simulink model "cllc_plant"  (R2020b)
settings: Solver=FixedStepDiscrete  StartTime=0.0  StopTime=Inf  FixedStep=stepsize  RelTol=1e-3  EnableMultiTasking=on
values from neighbouring files (symbols this model uses):
  Lm1 = Ln*LrP1    (= 0.00016)    [CLLC_Plant_Parameters.m]
  n = 20.0/9.0    (= 2.22222222222)    [CLLC_Plant_Parameters.m]
  stepsize = 2.0E-7    [cllc_data_lib.sldd]
  var_dir_v2g = 0.0    [cllc_data_lib.sldd]
  var_ref_iout = 18.5    [cllc_data_lib.sldd]
  var_ref_vout = 250.0    [cllc_data_lib.sldd]
libraries: fl_lib x219, ee_lib x151, nesl_utility x117, powerlib_meascontrol x15, eeStairGenerator x1
(part 1 of 8)
settings Model: DataDictionary=cllc_data_lib.sldd  ExtModeTrigDuration=8  Creator=wanikmalwansulami  LastModifiedBy=sgcesuser2
settings SolverCC: AutoInsertRateTranBlk=on  InsertRTBMode=Always
settings DataIOCC: SaveOutput=off  SaveTime=off  ReturnWorkspaceOutputs=off
settings OptimizationCC: DefaultUnderspecifiedDataType=single  EnhancedBackFolding=on  PassReuseOutputArgsAs=Individual arguments  MaxStackSize=1024  OptimizeBlockOrder=speed  DifferentSizesBufferReuse=on  OptimizationCustomize=off  DenormalBehavior=FlushToZero  EfficientTunableParamExpr=on
settings DebuggingCC: ParameterTunabilityLossMsg=error
settings HardwareCC: ProdBitPerChar=16  ProdBitPerInt=16  ProdBitPerPointer=32  ProdBitPerSizeT=32  ProdBitPerPtrDiffT=32  ProdLargestAtomicInteger=Integer  ProdLargestAtomicFloat=None  ProdWordSize=16  ProdLongLongMode=on  ProdHWDeviceType=Texas Instruments->C2000
settings SFSimCC: MATLABDynamicMemAlloc=off  CustomCodeUndefinedFunction=UseInterfaceOnly
settings RTWCC: Description=Embedded Coder  SystemTargetFile=ert.tlc  HardwareBoard=TI Piccolo F2807x  TemplateMakefile=ert_default_tmf  Toolchain=Texas Instruments Code Composer Studio (C2000)  PortableWordSizes=on
settings CodeAppCC: ForceParamTrailComments=on  IgnoreCustomStorageClasses=off  OperatorAnnotations=on  SimulinkDataObjDesc=on  SFDataObjDesc=on  InsertBlockDesc=on
settings ERTTargetCC: CodeReplacementLibrary=TI C28x  CombineOutputUpdateFcns=off  SupportContinuousTime=on  SupportNonInlinedSFcns=on  ExtModeStaticAllocSize=2000
settings SimscapeCC: SimscapeLogSimulationStatistics=on  SimscapeLogLimitData=off

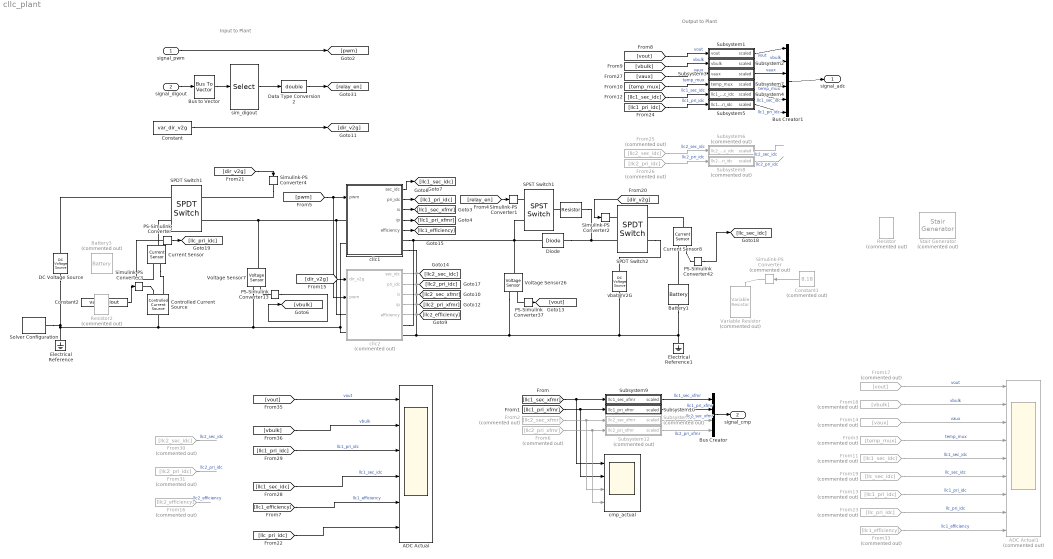
== system cllc_plant ==
  note: Input to Plant
  note: Output to Plant
  signal_pwm : Inport
  signal_digout : Inport  Port=2
  " " : ee_lib/Passive/Resistor  R=0.5e-3 Ohm  R_tol=1  enable_R_tol=0  tol_distribution=1  nSigma=4  enable_operating_limits=0  operating_limit_action=2  max_working_voltage=100 V  power_rating=1 W  enable_faults=0  fault_action=1  R_faulted=inf Ohm  enable_temporal_fault=0  t_fault=1 s  enable_behavioral_fault=0  max_permissible_current=1 A  t_fail_on_current=1 s  noise_mode=0  sample_time=1e-3 s  repeatability=1  auto_seed=988016956  user_seed=0  Tdevice=25 degC  alpha=3.93e-3 1/K  Tmeas=25 degC  thermal_mass=100 J/K  power_derating_T1=70 degC  power_derating_T2=155 degC  operating_temperature_range_vec=[-50, 150] degC  temperature_specify=off  temperature_priority=High  temperature=298.15 K  temperature_nominal_specify=off  temperature_nominal_unit=K  temperature_nominal_value=1
  ADC Actual : Scope  NumInputPorts=6
  ADC Actual1 : Scope  Commented=on  NumInputPorts=9
  Battery1 : ee_lib/Sources/Battery  Vnom=var_ref_vout V  prm_dir=1  R1_dis=2 Ohm  R1_ch=2 Ohm  R1=1e-3 Ohm  prm_AH=2  AH=(10*var_ref_iout)/3.6e6 hr*A  V1=var_ref_vout*0.1 V  AH1=0.1/3.6e6 hr*A  prm_R2=1  R2=2000 Ohm  prm_dyn=1  Rp1=0.005 Ohm  tau1=1 hr  Rp2=0.005 Ohm  tau2=30 s  Rp3=0.005 Ohm  tau3=30 s  Rp4=0.005 Ohm  tau4=30 s  Rp5=0.005 Ohm  tau5=30 s  prm_fade=1  N_fade=100  AH_fade=45 hr*A  R1_fade=2.02 Ohm  R1_ch_fade=2.02 Ohm  V1_fade=10.35 V  i_specify=off  i_priority=None  i=0 A  i_nominal_specify=off  i_nominal_unit=A  i_nominal_value=1  v_specify=on  v_priority=None  v=var_ref_vout*0.1 V  v_nominal_specify=off  v_nominal_unit=V  v_nominal_value=1  charge_specify=on  charge_priority=High  charge=0.1/3.6e6 hr*A  charge_nominal_specify=off  charge_nominal_unit=hr*A  charge_nominal_value=1  num_cycles_specify=off  num_cycles_priority=High  num_cycles=0  num_cycles_nominal_specify=off  num_cycles_nominal_unit=1  num_cycles_nominal_value=1  thermal_mass=30000 J/K  Tmeas=298.15 K  Vnom_T2=12 V  R1_T2=2.2 Ohm  R1_T2_dis=2.2 Ohm  R1_T2_ch=2.2 Ohm  V1_T2=11.4 V  R2_T2=2200 Ohm  Rp1_T2=0.005 Ohm  tau1_T2=30 s  Rp2_T2=0.005 Ohm  tau2_T2=30 s  Rp3_T2=0.005 Ohm  tau3_T2=30 s  Rp4_T2=0.005 Ohm  tau4_T2=30 s  Rp5_T2=0.005 Ohm  tau5_T2=30 s  Tmeas2=273.15 K  temperature_specify=off  temperature_priority=High  temperature=298.15 K  temperature_nominal_specify=off  temperature_nominal_unit=K  temperature_nominal_value=1
  Battery3 : ee_lib/Sources/Battery  Commented=on  Vnom=800 V  prm_dir=1  R1_dis=2 Ohm  R1_ch=2 Ohm  R1=1e-3 Ohm  prm_AH=2  AH=(10*var_ref_iout)/3.6e6 hr*A  V1=800*0.1 V  AH1=0.1/3.6e6 hr*A  prm_R2=1  R2=2000 Ohm  prm_dyn=1  Rp1=0.005 Ohm  tau1=1 hr  Rp2=0.005 Ohm  tau2=30 s  Rp3=0.005 Ohm  tau3=30 s  Rp4=0.005 Ohm  tau4=30 s  Rp5=0.005 Ohm  tau5=30 s  prm_fade=1  N_fade=100  AH_fade=45 hr*A  R1_fade=2.02 Ohm  R1_ch_fade=2.02 Ohm  V1_fade=10.35 V  i_specify=off  i_priority=None  i=0 A  i_nominal_specify=off  i_nominal_unit=A  i_nominal_value=1  v_specify=on  v_priority=None  v=var_ref_vout*0.1 V  v_nominal_specify=off  v_nominal_unit=V  v_nominal_value=1  charge_specify=on  charge_priority=High  charge=0.1/3.6e6 hr*A  charge_nominal_specify=off  charge_nominal_unit=hr*A  charge_nominal_value=1  num_cycles_specify=off  num_cycles_priority=High  num_cycles=0  num_cycles_nominal_specify=off  num_cycles_nominal_unit=1  num_cycles_nominal_value=1  thermal_mass=30000 J/K  Tmeas=298.15 K  Vnom_T2=12 V  R1_T2=2.2 Ohm  R1_T2_dis=2.2 Ohm  R1_T2_ch=2.2 Ohm  V1_T2=11.4 V  R2_T2=2200 Ohm  Rp1_T2=0.005 Ohm  tau1_T2=30 s  Rp2_T2=0.005 Ohm  tau2_T2=30 s  Rp3_T2=0.005 Ohm  tau3_T2=30 s  Rp4_T2=0.005 Ohm  tau4_T2=30 s  Rp5_T2=0.005 Ohm  tau5_T2=30 s  Tmeas2=273.15 K  temperature_specify=off  temperature_priority=High  temperature=298.15 K  temperature_nominal_specify=off  temperature_nominal_unit=K  temperature_nominal_value=1
  Bus Creator : BusCreator  Inputs=4  OutDataTypeStr=Bus: signal_cmp
      settings: InheritFromInputs=off
  Bus Creator1 : BusCreator  Inputs=6  OutDataTypeStr=Bus: signal_adc
      settings: InheritFromInputs=off
  Bus to Vector : BusToVector
  Constant : Constant  Value=var_dir_v2g
  Constant1 : Constant  Commented=on  Value=8.18
  Constant2 : Constant  Value=var_ref_iout
  Controlled Current Source : fl_lib/Electrical/Electrical Sources/Controlled Current Source
  Current Sensor : fl_lib/Electrical/Electrical Sensors/Current Sensor
  Current Sensor8 : fl_lib/Electrical/Electrical Sensors/Current Sensor
  DC Voltage Source : fl_lib/Electrical/Electrical Sources/DC Voltage Source  v0=v_input V
  Data Type Conversion2 : DataTypeConversion  OutDataTypeStr=double
  Diode : ee_lib/Semiconductors & Converters/Diode  ModelType=ee.enum.diode.modelType.pwl  IfMat=[.07, .12, .19, 1.75, 4.24, 7.32, 11.2; .16, .3, .72, 2.14, 4.02, 6.35, 9.12] A  TjVec=[25, 125] degC  VfVec=[.5, .7, .9, 1.3, 1.7, 2.1, 2.5] V  Vf=0.6 V  Ron=0.3 Ohm  Goff=1e-8 S  prmExp=ee.enum.diode.expParam.useTwo  I12=[.0137, .545] A  V12=[.6, .7] V  IS=1e-12 A  ec=1  I1=0.0137 A  V1=0.6 V  RS=0 Ohm  Tmeas=25 degC  N_series=1  N_parallel=1  Rz=0.3 Ohm  BV=inf V  C_param=ee.enum.diode.capParam.fixed  CJ=5 pF  CJ0=5 pF  VJ=1 V  Mgrad=0.5  Vvec=[.1, 10, 100] V  Cvec=[3.5, 1, .4] pF  FC=0.5  Q_param=ee.enum.diode.recoveryParam.off  iRM=-7.15 A  iF=4 A  didt=-750 A/us  trr_factor=3  trr=115 ns  Qrr=1500 s*uA  TT=50 ns  tau=100 ns  T_param=ee.enum.diode.temperatureParam.off  IS_T2=1.25e-7 A  I1_T2=0.245 A  V1_T2=0.5 V  Tmeas2=125 degC  EG_param=ee.enum.diode.egapParam.material_si  EG=1.11 eV  XTI_param=ee.enum.diode.xtiParam.pn  XTI=3  dBVdT=0 V/K  Tdevice=25 degC  i_specify=off  i_priority=None  i=0 A  i_nominal_specify=off  i_nominal_unit=A  i_nominal_value=1  v_specify=off  v_priority=None  v=0 V  v_nominal_specify=off  v_nominal_unit=V  v_nominal_value=1  i_capacitor_specify=off  i_capacitor_priority=None  i_capacitor=0 A  i_capacitor_nominal_specify=off  i_capacitor_nominal_unit=A  i_capacitor_nominal_value=1  v_capacitor_specify=off  v_capacitor_priority=None  v_capacitor=0 V  v_capacitor_nominal_specify=off  v_capacitor_nominal_unit=V  v_capacitor_nominal_value=1  power_dissipated_specify=off  power_dissipated_priority=None  power_dissipated=0 W  power_dissipated_nominal_specify=off  power_dissipated_nominal_unit=W  power_dissipated_nominal_value=1  thermal_network_parameterization=ee.enum.thermalNetworkTopology.cauer  Rth=[0, 10] K/W  Rth_Foster=[4, 6] K/W  thermal_mass_parameterization=ee.enum.thermalNetwork.timeconstant  thermal_mass=[0, 1] J/K  thermal_mass_Foster=[1.5, 3] J/K  thermal_time_constant=[0, 10] s  thermal_time_constant_Foster=[6, 18] s  thermal_mass_initial_temperatures=[25, 25] degC
  Electrical Reference : fl_lib/Electrical/Electrical Elements/Electrical Reference
  Electrical Reference1 : fl_lib/Electrical/Electrical Elements/Electrical Reference
  From11 : From  Commented=on  GotoTag=llc1_sec_idc
  From13 : From  Commented=on  GotoTag=llc1_pri_idc
  From14 : From  Commented=on  GotoTag=vaux
  From16 : From  Commented=on  GotoTag=llc2_efficiency
  From17 : From  Commented=on  GotoTag=vout
  From18 : From  Commented=on  GotoTag=vbulk
  From19 : From  Commented=on  GotoTag=llc_sec_idc
  From2 : From  Commented=on  GotoTag=llc2_sec_xfmr
  From23 : From  Commented=on  GotoTag=llc_pri_idc
  From25 : From  Commented=on  GotoTag=llc2_sec_idc
  From26 : From  Commented=on  GotoTag=llc2_pri_idc
  From3 : From  Commented=on  GotoTag=temp_mux
  From30 : From  Commented=on  GotoTag=llc2_sec_idc
  From31 : From  Commented=on  GotoTag=llc2_pri_idc
  From33 : From  Commented=on  GotoTag=llc1_efficiency
  From6 : From  Commented=on  GotoTag=llc2_pri_xfmr
  PS-Simulink Converter : nesl_utility/PS-Simulink Converter  PhysicalDomain=network_engine_domain  SubClassName=ps_output  LeftPortType=input  RightPortType=output  PseudoPeriodic=off  Frequencies=[]  Unit=inherit  AffineConversion=off
  PS-Simulink Converter13 : nesl_utility/PS-Simulink Converter  PhysicalDomain=network_engine_domain  SubClassName=ps_output  LeftPortType=input  RightPortType=output  PseudoPeriodic=off  Frequencies=[]  Unit=1  AffineConversion=off
  PS-Simulink Converter37 : nesl_utility/PS-Simulink Converter  PhysicalDomain=network_engine_domain  SubClassName=ps_output  LeftPortType=input  RightPortType=output  PseudoPeriodic=off  Frequencies=[]  Unit=1  AffineConversion=off
  PS-Simulink Converter42 : nesl_utility/PS-Simulink Converter  PhysicalDomain=network_engine_domain  SubClassName=ps_output  LeftPortType=input  RightPortType=output  PseudoPeriodic=off  Frequencies=[]  Unit=1  AffineConversion=off
  Resistor : fl_lib/Electrical/Electrical Elements/Resistor  Commented=on  R=300*300/11000 Ohm  i_specify=off  i_priority=None  i=0 A  i_nominal_specify=off  i_nominal_unit=A  i_nominal_value=1  v_specify=off  v_priority=None  v=0 V  v_nominal_specify=off  v_nominal_unit=V  v_nominal_value=1
  Resistor2 : fl_lib/Electrical/Electrical Elements/Resistor  Commented=on  R=800/var_ref_iout Ohm  i_specify=off  i_priority=None  i=0 A  i_nominal_specify=off  i_nominal_unit=A  i_nominal_value=1  v_specify=off  v_priority=None  v=0 V  v_nominal_specify=off  v_nominal_unit=V  v_nominal_value=1
  SPDT Switch1 : ee_lib/Switches & Breakers/SPDT Switch  R_closed=0.01 Ohm  G_open=1e-6 S  Threshold=0.5 V  Width=0 V  model_dynamics=0  t_on=1e-3 s  t_off=1e-3 s  initial_vT=0 V
      settings: SourceProductBaseCode=PS
  SPDT Switch2 : ee_lib/Switches & Breakers/SPDT Switch  R_closed=0.01 Ohm  G_open=1e-6 S  Threshold=0.5 V  Width=0 V  model_dynamics=0  t_on=1e-3 s  t_off=1e-3 s  initial_vT=0 V
      settings: SourceProductBaseCode=PS
  SPST Switch1 : ee_lib/Switches & Breakers/SPST Switch  R_closed=0.01 Ohm  G_open=1e-6 S  Threshold=0.5 V  Width=0 V  model_dynamics=0  t_on=1e-3 s  t_off=1e-3 s  initial_vT=0 V
      settings: SourceProductBaseCode=PS  InternalSimscapePortConfiguration="{\"Bottom\":[],\"Left\":[{\"id\":\"vT\",\"label\":\"vT\",\"type\":\"input\"},{\"id\":\"p\",\"label\":\"\",\"type\":\"foundation.electrical.electrical\"}],\"Right\":[{\"id\":\"n\",\"label\":\"\",\"type\":\"foundation.electrical.electrical\"}],\"Top\":[]}"
  Simulink-PS Converter : nesl_utility/Simulink-PS Converter  Commented=on  PhysicalDomain=network_engine_domain  SubClassName=ps_input  LeftPortType=input  RightPortType=output  PseudoPeriodic=off  Frequencies=[]  NoiseDistribution=none  NoiseParameters=[]  Unit=1  AffineConversion=off  FilteringAndDerivatives=provide  SimscapeFilterOrder=1  InputFilterTimeConstant=0.001  UdotUserProvided=0
  Simulink-PS Converter{1..4} (4 alike) : nesl_utility/Simulink-PS Converter  PhysicalDomain=network_engine_domain  SubClassName=ps_input  LeftPortType=input  RightPortType=output  PseudoPeriodic=off  Frequencies=[]  NoiseDistribution=none  NoiseParameters=[]  Unit=1  AffineConversion=off  FilteringAndDerivatives=provide  SimscapeFilterOrder=1  InputFilterTimeConstant=0.001  UdotUserProvided=0
  Solver Configuration : nesl_utility/Solver Configuration  PhysicalDomain=network_engine_domain  SubClassName=solver  LeftPortType=input  RightPortType=generic  Tones=[]  Harmonics=[]  SimulateNoise=off  Profile=off  UseLocalSampling=off  EnableSwitchedLinearOptims=on  FrequencyDomain=off  UseCCode=off  RelTol=0.001  AbsTol=1e-06  MinStep=1e-09  ToWorkspace=off  RevertToSquareIcSolve=off  NumHomotopyIterations=100  PhasorMode=off  PhasorModeNumHarmonics=1  DoDC=off  ResidualTolerance=stepsize  UseLocalSolver=on  LocalSolverChoice=NE_BACKWARD_EULER_ADVANCER  LocalSolverSampleTime=stepsize  DoFixedCost=off  MaxNonlinIter=3  MaxModeIter=2  ComputeImpulses=off  ImpulseIterations=2  LinearAlgebra=auto  EquationFormulation=NE_TIME_EF  DelaysMemoryBudget=1024  AutomaticFiltering=on  FilteringTimeConstant=0.001  PartitionStorageMethod=AS_NEEDED  PartitionMemoryBudget=1024  PartitionMethod=FAST
  Stair Generator : eeStairGenerator/Stair Generator  Commented=on  LabelModeActiveChoice=Discrete  TimeInput=[0 1]  AmplitudeInput="[8.18  3]"  SampleTime=-1  RepeatPattern=off  OutDataTypeStr=double
      settings: SourceProductBaseCode=PS
  Subsystem1 : Subsystem
  Subsystem10 : Subsystem
  Subsystem11 : Subsystem  Commented=on
  Subsystem12 : Subsystem  Commented=on
  Subsystem2 : Subsystem
  Subsystem3 : Subsystem
  Subsystem4 : Subsystem
  Subsystem5 : Subsystem
  Subsystem6 : Subsystem  Commented=on
  Subsystem7 : Subsystem
  Subsystem8 : Subsystem  Commented=on
  Subsystem9 : Subsystem
  Variable Resistor : fl_lib/Electrical/Electrical Elements/Variable Resistor  Commented=on  Rmin=8.18 Ohm  i_specify=off  i_priority=None  i=0 A  i_nominal_specify=off  i_nominal_unit=A  i_nominal_value=1  v_specify=off  v_priority=None  v=0 V  v_nominal_specify=off  v_nominal_unit=V  v_nominal_value=1
  Voltage Sensor26 : fl_lib/Electrical/Electrical Sensors/Voltage Sensor
  Voltage Sensor7 : fl_lib/Electrical/Electrical Sensors/Voltage Sensor
  cllc1 : Subsystem
  cllc2 : Subsystem  Commented=on
  cmp_actual : Scope  NumInputPorts=4
  sim_digout : Selector  InputPortWidth=10  IndexOptions=Index vector (dialog)  Indices=[10]  OutputSizes=1
  vbat@V2G : fl_lib/Electrical/Electrical Sources/DC Voltage Source  v0=var_ref_vout V
  signal_adc : Outport  OutDataTypeStr=Bus: signal_adc  BusOutputAsStruct=on
  signal_cmp : Outport  Port=2  OutDataTypeStr=Bus: signal_cmp
  wires:
  [pwm] -> cllc2/2(pwm), cllc1/1(pwm)
  PS-Simulink Converter37/1 -> [vout]
  PS-Simulink Converter13/1 -> [vbulk]
  [dir_v2g] -> Simulink-PS Converter4/1
  [relay_en] -> Simulink-PS Converter1/1
  cllc1/3(is) -> [llc1_sec_xfmr]
  [vout] -> Subsystem1/1(vout)  "vout"
  [vbulk] -> Subsystem2/1(vbulk)  "vbulk"
  [vaux] -> Subsystem3/1(vaux)  "vaux"
  [temp_mux] -> Subsystem7/1(temp_mux)  "temp_mux"
  [llc1_sec_idc] -> Subsystem4/1(llc1_sec_idc)  "llc1_sec_idc"
  [llc1_pri_idc] -> Subsystem5/1(llc1_pri_idc)  "llc1_pri_idc"
  From25/1 -> Subsystem6/1(llc2_sec_idc)  "llc2_sec_idc"
  From26/1 -> Subsystem8/1(llc2_pri_idc)  "llc2_pri_idc"
  Subsystem1/1(scaled) -> Bus Creator1/1  "vout"
  Subsystem2/1(scaled) -> Bus Creator1/2  "vbulk"
  Subsystem3/1(scaled) -> Bus Creator1/3  "vaux"
  Subsystem7/1(scaled) -> Bus Creator1/4  "temp_mux"
  Subsystem4/1(scaled) -> Bus Creator1/5  "llc1_sec_idc"
  Subsystem5/1(scaled) -> Bus Creator1/6  "llc1_pri_idc"
  Subsystem6/1(scaled) -> ?  "llc2_sec_idc"
  Subsystem8/1(scaled) -> ?  "llc2_pri_idc"
  Bus Creator1/1 -> signal_adc/1
  cllc1/1(sec_idc) -> [llc1_sec_idc]
  cllc1/2(pri_idc) -> [llc1_pri_idc]
  cllc1/4(ip) -> [llc1_pri_xfmr]
  [llc1_sec_xfmr] -> cmp_actual/1, Subsystem9/1(llc1_sec_xfmr)
  [llc1_pri_xfmr] -> cmp_actual/2, Subsystem10/1(llc1_pri_xfmr)
  From2/1 -> cmp_actual/3, Subsystem11/1(llc2_sec_xfmr)
  From6/1 -> cmp_actual/4, Subsystem12/1(llc2_pri_xfmr)
  Subsystem9/1(scaled) -> Bus Creator/1  "llc1_sec_xfmr"
  Subsystem10/1(scaled) -> Bus Creator/2  "llc1_pri_xfmr"
  Subsystem11/1(scaled) -> Bus Creator/3  "llc2_sec_xfmr"
  Subsystem12/1(scaled) -> Bus Creator/4  "llc2_pri_xfmr"
  Bus Creator/1 -> signal_cmp/1
  [llc1_efficiency] -> ADC Actual/5  "llc1_efficiency"
  From16/1 -> ?  "llc2_efficiency"
  cllc1/5(efficiency) -> [llc1_efficiency]
  [dir_v2g] -> Simulink-PS Converter2/1
  PS-Simulink Converter/1 -> [llc_pri_idc]
  signal_pwm/1 -> [pwm]
  cllc2/5(efficiency) -> [llc2_efficiency]
  cllc2/1(sec_idc) -> [llc2_sec_idc]
  cllc2/2(pri_idc) -> [llc2_pri_idc]
  cllc2/3(is) -> [llc2_sec_xfmr]
  cllc2/4(ip) -> [llc2_pri_xfmr]
  PS-Simulink Converter42/1 -> [llc_sec_idc]
  [vout] -> ADC Actual/1  "vout"
  [vbulk] -> ADC Actual/2  "vbulk"
  [llc1_sec_idc] -> ADC Actual/4  "llc1_sec_idc"
  From30/1 -> ?  "llc2_sec_idc"
  [llc1_pri_idc] -> ADC Actual/3  "llc1_pri_idc"
  From31/1 -> ?  "llc2_pri_idc"
  [dir_v2g] -> cllc2/1(dir_v2g)
  sim_digout/1 -> Data Type Conversion2/1
  Bus to Vector/1 -> sim_digout/1
  signal_digout/1 -> Bus to Vector/1
  Data Type Conversion2/1 -> [relay_en]
  Constant/1 -> [dir_v2g]
  From17/1 -> ADC Actual1/1  "vout"
  From19/1 -> ADC Actual1/6  "llc_sec_idc"
  From23/1 -> ADC Actual1/8  "llc_pri_idc"
  From18/1 -> ADC Actual1/2  "vbulk"
  From33/1 -> ADC Actual1/9  "llc1_efficiency"
  From14/1 -> ADC Actual1/3  "vaux"
  From13/1 -> ADC Actual1/7  "llc1_pri_idc"
  From11/1 -> ADC Actual1/5  "llc1_sec_idc"
  From3/1 -> ADC Actual1/4  "temp_mux"
  Constant1/1 -> Simulink-PS Converter/1
  [llc_pri_idc] -> ADC Actual/6
  Constant2/1 -> Simulink-PS Converter3/1
  connections:
  PS-Simulink Converter13/LConn1 -- Voltage Sensor7/RConn1
  PS-Simulink Converter37/LConn1 -- Voltage Sensor26/RConn1
  Battery1/RConn1 -- Electrical Reference1/LConn1 -- vbat@V2G/RConn1 -- Voltage Sensor26/RConn2 -- cllc2/RConn2 -- cllc1/RConn2
  Simulink-PS Converter4/RConn1 -- SPDT Switch1/LConn1
  DC Voltage Source/LConn1 -- SPDT Switch1/RConn1
  SPDT Switch2/RConn2 -- vbat@V2G/LConn1
  Diode/RConn1 -- " "/RConn1 -- SPDT Switch2/LConn2
  SPST Switch1/LConn1 -- Simulink-PS Converter1/RConn1
  Solver Configuration/RConn1 -- DC Voltage Source/RConn1 -- Electrical Reference/LConn1 -- Controlled Current Source/LConn1 -- Voltage Sensor7/RConn2 -- cllc1/LConn2 -- cllc2/LConn2
  Simulink-PS Converter2/RConn1 -- SPDT Switch2/LConn1
  SPDT Switch1/RConn2 -- Current Sensor/LConn1
  Current Sensor/RConn2 -- Controlled Current Source/RConn2
  PS-Simulink Converter/LConn1 -- Current Sensor/RConn1
  Battery1/LConn1 -- Current Sensor8/RConn2
  Current Sensor8/RConn1 -- PS-Simulink Converter42/LConn1
  Current Sensor8/LConn1 -- SPDT Switch2/RConn1
  cllc2/LConn1 -- SPDT Switch1/LConn2 -- Voltage Sensor7/LConn1 -- cllc1/LConn1
  SPST Switch1/RConn1 -- " "/LConn1
  SPST Switch1/LConn2 -- cllc2/RConn1 -- cllc1/RConn1 -- Diode/LConn1 -- Voltage Sensor26/LConn1
  Simulink-PS Converter/RConn1 -- Variable Resistor/LConn1
  Simulink-PS Converter3/RConn1 -- Controlled Current Source/RConn1

== system cllc_plant/Subsystem1 ==
  note: Analog filter:
      | fc = 159kHz
      | R = 1kOhm
      | C = 1nF
  note: Hardware
      | Scaling
  vout : Inport
  Data Type Conversion6 : DataTypeConversion  OutDataTypeStr=single
  First-Order Filter1 : powerlib_meascontrol/Filters/First-Order Filter  Commented=on  FilterType=Lowpass  Tc=10e-6  Ts=0  Initialize=off  Vac_Init=[0, 0, 60]  Vdc_Init=0  PlotResponse=off  FreqRange="[0,  200,  1]"
  Gain2 : Gain  Gain=0.0056659
  Random Number2 : RandomNumber  Commented=on  Variance=100  Seed=3  SampleTime=0
  Sum2 : Sum  Inputs=|++
  scaled : Outport
  wires:
  Data Type Conversion6/1 -> scaled/1
  Sum2/1 -> Gain2/1
  Random Number2/1 -> Sum2/2
  Gain2/1 -> Data Type Conversion6/1
  vout/1 -> Sum2/1

== system cllc_plant/Subsystem10 ==
  note: Hardware
      | Scaling
  note: Analog filter:
      | fc = 159kHz
      | R = 1kOhm
      | C = 1nF
  llc1_pri_xfmr : Inport
  Data Type Conversion6 : DataTypeConversion  OutDataTypeStr=single
  First-Order Filter1 : powerlib_meascontrol/Filters/First-Order Filter  Commented=on  FilterType=Lowpass  Tc=10e-6  Ts=0  Initialize=off  Vac_Init=[0, 0, 60]  Vdc_Init=0  PlotResponse=off  FreqRange="[0,  200,  1]"
  Gain2 : Gain
  Random Number2 : RandomNumber  Commented=on  Variance=100  Seed=3  SampleTime=0
  Sum2 : Sum  Inputs=|++
  scaled : Outport
  wires:
  llc1_pri_xfmr/1 -> Sum2/1
  Gain2/1 -> Data Type Conversion6/1
  Random Number2/1 -> Sum2/2
  Sum2/1 -> Gain2/1
  Data Type Conversion6/1 -> scaled/1

== system cllc_plant/Subsystem11 ==
  note: Analog filter:
      | fc = 159kHz
      | R = 1kOhm
      | C = 1nF
  note: Hardware
      | Scaling
  llc2_sec_xfmr : Inport
  Data Type Conversion6 : DataTypeConversion  OutDataTypeStr=single
  First-Order Filter1 : powerlib_meascontrol/Filters/First-Order Filter  Commented=on  FilterType=Lowpass  Tc=10e-6  Ts=0  Initialize=off  Vac_Init=[0, 0, 60]  Vdc_Init=0  PlotResponse=off  FreqRange="[0,  200,  1]"
  Gain2 : Gain
  Random Number2 : RandomNumber  Commented=on  Variance=100  Seed=3  SampleTime=0
  Sum2 : Sum  Inputs=|++
  scaled : Outport
  wires:
  Data Type Conversion6/1 -> scaled/1
  Sum2/1 -> Gain2/1
  Random Number2/1 -> Sum2/2
  Gain2/1 -> Data Type Conversion6/1
  llc2_sec_xfmr/1 -> Sum2/1

== system cllc_plant/Subsystem12 ==
  note: Hardware
      | Scaling
  note: Analog filter:
      | fc = 159kHz
      | R = 1kOhm
      | C = 1nF
  llc2_pri_xfmr : Inport
  Data Type Conversion6 : DataTypeConversion  OutDataTypeStr=single
  First-Order Filter1 : powerlib_meascontrol/Filters/First-Order Filter  Commented=on  FilterType=Lowpass  Tc=10e-6  Ts=0  Initialize=off  Vac_Init=[0, 0, 60]  Vdc_Init=0  PlotResponse=off  FreqRange="[0,  200,  1]"
  Gain2 : Gain
  Random Number2 : RandomNumber  Commented=on  Variance=100  Seed=3  SampleTime=0
  Sum2 : Sum  Inputs=|++
  scaled : Outport
  wires:
  llc2_pri_xfmr/1 -> Sum2/1
  Gain2/1 -> Data Type Conversion6/1
  Random Number2/1 -> Sum2/2
  Sum2/1 -> Gain2/1
  Data Type Conversion6/1 -> scaled/1

== system cllc_plant/Subsystem2 ==
  note: Hardware
      | Scaling
  note: Analog filter:
      | fc = 159kHz
      | R = 1kOhm
      | C = 1nF
  vbulk : Inport
  Data Type Conversion6 : DataTypeConversion  OutDataTypeStr=single
  First-Order Filter1 : powerlib_meascontrol/Filters/First-Order Filter  Commented=on  FilterType=Lowpass  Tc=10e-6  Ts=0  Initialize=off  Vac_Init=[0, 0, 60]  Vdc_Init=0  PlotResponse=off  FreqRange="[0,  200,  1]"
  Gain1 : Gain  Gain=0.0036102
  Random Number2 : RandomNumber  Commented=on  Variance=100  Seed=3  SampleTime=0
  Sum2 : Sum  Inputs=|++
  scaled : Outport
  wires:
  vbulk/1 -> Sum2/1
  Gain1/1 -> Data Type Conversion6/1
  Random Number2/1 -> Sum2/2
  Sum2/1 -> Gain1/1
  Data Type Conversion6/1 -> scaled/1

== system cllc_plant/Subsystem3 ==
  note: Analog filter:
      | fc = 159kHz
      | R = 1kOhm
      | C = 1nF
  note: Hardware
      | Scaling
  vaux : Inport
  Data Type Conversion6 : DataTypeConversion  OutDataTypeStr=single
  First-Order Filter1 : powerlib_meascontrol/Filters/First-Order Filter  Commented=on  FilterType=Lowpass  Tc=10e-6  Ts=0  Initialize=off  Vac_Init=[0, 0, 60]  Vdc_Init=0  PlotResponse=off  FreqRange="[0,  200,  1]"
  Gain2 : Gain  Gain=0.0036102
  Random Number2 : RandomNumber  Commented=on  Variance=100  Seed=3  SampleTime=0
  Sum2 : Sum  Inputs=|++
  scaled : Outport
  wires:
  Data Type Conversion6/1 -> scaled/1
  Sum2/1 -> Gain2/1
  Random Number2/1 -> Sum2/2
  Gain2/1 -> Data Type Conversion6/1
  vaux/1 -> Sum2/1

== system cllc_plant/Subsystem4 ==
  note: Hardware
      | Scaling
  note: Analog filter:
      | fc = 159kHz
      | R = 1kOhm
      | C = 1nF
  llc1_sec_idc : Inport
  Data Type Conversion6 : DataTypeConversion  OutDataTypeStr=single
  First-Order Filter1 : powerlib_meascontrol/Filters/First-Order Filter  Commented=on  FilterType=Lowpass  Tc=10e-6  Ts=0  Initialize=off  Vac_Init=[0, 0, 60]  Vdc_Init=0  PlotResponse=off  FreqRange="[0,  200,  1]"
  Gain1 : Gain  Commented=on  Gain=0.0269
  Gain2 : Gain  Gain=20e-3
  Random Number2 : RandomNumber  Commented=on  Variance=100  Seed=3  SampleTime=0
  Sum2 : Sum  Inputs=|++
  scaled : Outport
  wires:
  llc1_sec_idc/1 -> Sum2/1
  Gain2/1 -> Data Type Conversion6/1
  Random Number2/1 -> Sum2/2
  Sum2/1 -> Gain2/1
  Data Type Conversion6/1 -> scaled/1

== system cllc_plant/Subsystem5 ==
  note: Gain calculation:
      | Parallel res: 1e-3
      | AMC: 8.2
      | Diff amp: 22.1/1.5
  note: Analog filter:
      | fc = 159kHz
      | R = 1kOhm
      | C = 1nF
  note: Hardware
      | Scaling
  llc1_pri_idc : Inport
  Data Type Conversion6 : DataTypeConversion  OutDataTypeStr=single
  First-Order Filter1 : powerlib_meascontrol/Filters/First-Order Filter  Commented=on  FilterType=Lowpass  Tc=10e-6  Ts=0  Initialize=off  Vac_Init=[0, 0, 60]  Vdc_Init=0  PlotResponse=off  FreqRange="[0,  200,  1]"
  Gain2 : Gain  Gain=0.1208
  Random Number2 : RandomNumber  Commented=on  Variance=100  Seed=3  SampleTime=0
  Sum2 : Sum  Inputs=|++
  scaled : Outport
  wires:
  Data Type Conversion6/1 -> scaled/1
  Sum2/1 -> Gain2/1
  Random Number2/1 -> Sum2/2
  Gain2/1 -> Data Type Conversion6/1
  llc1_pri_idc/1 -> Sum2/1

== system cllc_plant/Subsystem6 ==
  note: Hardware
      | Scaling
  note: Analog filter:
      | fc = 159kHz
      | R = 1kOhm
      | C = 1nF
  note: Gain calculation:
      | Parallel res: 1e-3
      | AMC: 8.2
      | Diff amp: 22.1/1.5
  llc2_sec_idc : Inport
  Data Type Conversion6 : DataTypeConversion  OutDataTypeStr=single
  First-Order Filter1 : powerlib_meascontrol/Filters/First-Order Filter  Commented=on  FilterType=Lowpass  Tc=10e-6  Ts=0  Initialize=off  Vac_Init=[0, 0, 60]  Vdc_Init=0  PlotResponse=off  FreqRange="[0,  200,  1]"
  Gain2 : Gain  Gain=0.1208
  Random Number2 : RandomNumber  Commented=on  Variance=100  Seed=3  SampleTime=0
  Sum2 : Sum  Inputs=|++
  scaled : Outport
  wires:
  llc2_sec_idc/1 -> Sum2/1
  Gain2/1 -> Data Type Conversion6/1
  Random Number2/1 -> Sum2/2
  Sum2/1 -> Gain2/1
  Data Type Conversion6/1 -> scaled/1

== system cllc_plant/Subsystem7 ==
  note: Hardware
      | Scaling
  note: Analog filter:
      | fc = 159kHz
      | R = 1kOhm
      | C = 1nF
  temp_mux : Inport
  Data Type Conversion6 : DataTypeConversion  OutDataTypeStr=single
  First-Order Filter1 : powerlib_meascontrol/Filters/First-Order Filter  Commented=on  FilterType=Lowpass  Tc=10e-6  Ts=0  Initialize=off  Vac_Init=[0, 0, 60]  Vdc_Init=0  PlotResponse=off  FreqRange="[0,  200,  1]"
  Gain2 : Gain  Gain=0.0036102
  Random Number2 : RandomNumber  Commented=on  Variance=100  Seed=3  SampleTime=0
  Sum2 : Sum  Inputs=|++
  scaled : Outport
  wires:
  temp_mux/1 -> Sum2/1
  Gain2/1 -> Data Type Conversion6/1
  Random Number2/1 -> Sum2/2
  Sum2/1 -> Gain2/1
  Data Type Conversion6/1 -> scaled/1

== system cllc_plant/Subsystem8 ==
  note: Analog filter:
      | fc = 159kHz
      | R = 1kOhm
      | C = 1nF
  note: Hardware
      | Scaling
  note: Gain calculation:
      | Parallel res: 1e-3
      | AMC: 8.2
      | Diff amp: 22.1/1.5
  llc2_pri_idc : Inport
  Data Type Conversion6 : DataTypeConversion  OutDataTypeStr=single
  First-Order Filter1 : powerlib_meascontrol/Filters/First-Order Filter  Commented=on  FilterType=Lowpass  Tc=10e-6  Ts=0  Initialize=off  Vac_Init=[0, 0, 60]  Vdc_Init=0  PlotResponse=off  FreqRange="[0,  200,  1]"
  Gain2 : Gain  Gain=0.1208
  Random Number2 : RandomNumber  Commented=on  Variance=100  Seed=3  SampleTime=0
  Sum2 : Sum  Inputs=|++
  scaled : Outport
  wires:
  Data Type Conversion6/1 -> scaled/1
  Sum2/1 -> Gain2/1
  Random Number2/1 -> Sum2/2
  Gain2/1 -> Data Type Conversion6/1
  llc2_pri_idc/1 -> Sum2/1

== system cllc_plant/Subsystem9 ==
  note: Analog filter:
      | fc = 159kHz
      | R = 1kOhm
      | C = 1nF
  note: Hardware
      | Scaling
  llc1_sec_xfmr : Inport
  Data Type Conversion6 : DataTypeConversion  OutDataTypeStr=single
  First-Order Filter1 : powerlib_meascontrol/Filters/First-Order Filter  Commented=on  FilterType=Lowpass  Tc=10e-6  Ts=0  Initialize=off  Vac_Init=[0, 0, 60]  Vdc_Init=0  PlotResponse=off  FreqRange="[0,  200,  1]"
  Gain2 : Gain
  Random Number2 : RandomNumber  Commented=on  Variance=100  Seed=3  SampleTime=0
  Sum2 : Sum  Inputs=|++
  scaled : Outport
  wires:
  Data Type Conversion6/1 -> scaled/1
  Sum2/1 -> Gain2/1
  Random Number2/1 -> Sum2/2
  Gain2/1 -> Data Type Conversion6/1
  llc1_sec_xfmr/1 -> Sum2/1

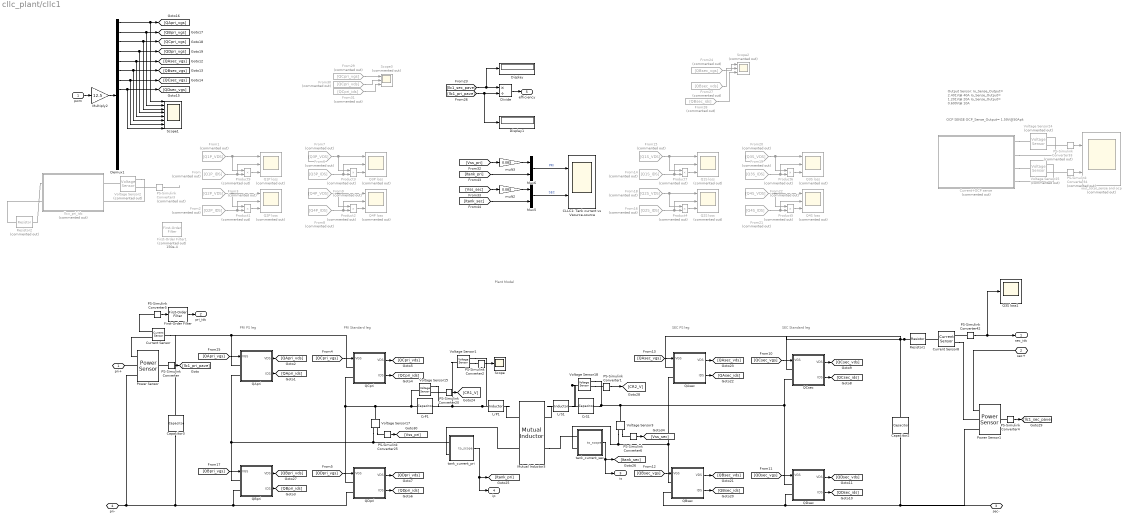
== system cllc_plant/cllc1 ==
  note: Plant Model
  note: 150e-4
  note: PRI PS leg
  note: Output Sensor:
      | Io_Sense_Output= 2.401V@ 40A
      | Io_Sense_Output= 1.201V@ 20A
      | Io_Sense_Output= 0.600V@ 10A
  note: OCP SENSE
      |
      | OCP_Sense_Output= 1.59V@50Apk
  note: PRI Standard leg
  note: SEC Standard leg
  note: SEC PS leg
  pwm : Inport
  CLLC1: Tank current vs Vsource-source : Scope  NumInputPorts=2
  Capacitor2 : fl_lib/Electrical/Electrical Elements/Capacitor  c=50e-6 F  r=9.5e-3 Ohm  g=0 1/Ohm  i_specify=off  i_priority=None  i=0 A  i_nominal_specify=off  i_nominal_unit=A  i_nominal_value=1  v_specify=off  v_priority=None  v=200 V  v_nominal_specify=off  v_nominal_unit=V  v_nominal_value=1  vc_specify=off  vc_priority=High  vc=0 V  vc_nominal_specify=off  vc_nominal_unit=V  vc_nominal_value=1
  Capacitor3 : fl_lib/Electrical/Electrical Elements/Capacitor  c=50e-6 F  r=9.4e-3 Ohm  g=0 1/Ohm  i_specify=off  i_priority=None  i=0 A  i_nominal_specify=off  i_nominal_unit=A  i_nominal_value=1  v_specify=on  v_priority=None  v=200 V  v_nominal_specify=off  v_nominal_unit=V  v_nominal_value=1  vc_specify=off  vc_priority=High  vc=0 V  vc_nominal_specify=off  vc_nominal_unit=V  vc_nominal_value=1
  CrP1 : fl_lib/Electrical/Electrical Elements/Capacitor  c=CrP1 F  r=1e-6 Ohm  g=0 1/Ohm  i_specify=off  i_priority=None  i=0 A  i_nominal_specify=off  i_nominal_unit=A  i_nominal_value=1  v_specify=off  v_priority=None  v=0 V  v_nominal_specify=off  v_nominal_unit=V  v_nominal_value=1  vc_specify=off  vc_priority=High  vc=0 V  vc_nominal_specify=off  vc_nominal_unit=V  vc_nominal_value=1
  CrS1 : fl_lib/Electrical/Electrical Elements/Capacitor  c=CrS1 F  r=1e-6 Ohm  g=0 1/Ohm  i_specify=off  i_priority=None  i=0 A  i_nominal_specify=off  i_nominal_unit=A  i_nominal_value=1  v_specify=off  v_priority=None  v=0 V  v_nominal_specify=off  v_nominal_unit=V  v_nominal_value=1  vc_specify=off  vc_priority=High  vc=0 V  vc_nominal_specify=off  vc_nominal_unit=V  vc_nominal_value=1
  Current Sensor : fl_lib/Electrical/Electrical Sensors/Current Sensor
  Current Sensor8 : fl_lib/Electrical/Electrical Sensors/Current Sensor
  Current+OCP sense : Subsystem  Commented=on
  Demux1 : Demux  Outputs=16
  Display : Display
  Display1 : Display
  Divide : Product  Inputs=*/
  First-Order Filter : powerlib_meascontrol/Filters/First-Order Filter  FilterType=Lowpass  Tc=150e-4  Ts=stepsize  Initialize=off  Vac_Init=[0, 0, 60]  Vdc_Init=0  PlotResponse=off  FreqRange="[0,  200,  1]"
  First-Order Filter1 : powerlib_meascontrol/Filters/First-Order Filter  Commented=on  FilterType=Lowpass  Tc=80e-3  Ts=50e-9  Initialize=off  Vac_Init=[0, 0, 60]  Vdc_Init=0  PlotResponse=off  FreqRange="[0,  200,  1]"
  From : From  Commented=on  GotoTag=Q1P_IDS
  From1 : From  Commented=on  GotoTag=Q1P_VDS
  From14 : From  Commented=on  GotoTag=Q1S_IDS
  From15 : From  Commented=on  GotoTag=Q1S_VDS
  From16 : From  Commented=on  GotoTag=Q2S_IDS
  From18 : From  Commented=on  GotoTag=Q2S_VDS
  From19 : From  Commented=on  GotoTag=Q3S_IDS
  From2 : From  Commented=on  GotoTag=Q2P_IDS
  From20 : From  Commented=on  GotoTag=Q3S_VDS
  From21 : From  Commented=on  GotoTag=Q4S_IDS
  From22 : From  Commented=on  GotoTag=Q4S_VDS
  From24 : From  Commented=on  GotoTag=QBsec_vgs
  From27 : From  Commented=on  GotoTag=QBsec_vds
  From28 : From  Commented=on  GotoTag=QBsec_ids
  From29 : From  Commented=on  GotoTag=QCpri_vgs
  From3 : From  Commented=on  GotoTag=Q2P_VDS
  From30 : From  Commented=on  GotoTag=QCpri_vds
  From31 : From  Commented=on  GotoTag=QCpri_ids
  From6 : From  Commented=on  GotoTag=Q3P_IDS
  From7 : From  Commented=on  GotoTag=Q3P_VDS
  From8 : From  Commented=on  GotoTag=Q4P_IDS
  From9 : From  Commented=on  GotoTag=Q4P_VDS
  LrP1 : fl_lib/Electrical/Electrical Elements/Inductor  l=LrP1 H  r=15e-3 Ohm  g=1e-9 1/Ohm  i_specify=off  i_priority=None  i=0 A  i_nominal_specify=off  i_nominal_unit=A  i_nominal_value=1  v_specify=off  v_priority=None  v=0 V  v_nominal_specify=off  v_nominal_unit=V  v_nominal_value=1  i_L_specify=off  i_L_priority=High  i_L=0 A  i_L_nominal_specify=off  i_L_nominal_unit=A  i_L_nominal_value=1
  LrS1 : fl_lib/Electrical/Electrical Elements/Inductor  l=LrS1 H  r=15e-3 Ohm  g=1e-9 1/Ohm  i_specify=off  i_priority=None  i=0 A  i_nominal_specify=off  i_nominal_unit=A  i_nominal_value=1  v_specify=off  v_priority=None  v=0 V  v_nominal_specify=off  v_nominal_unit=V  v_nominal_value=1  i_L_specify=off  i_L_priority=High  i_L=0 A  i_L_nominal_specify=off  i_L_nominal_unit=A  i_L_nominal_value=1
  Multiply2 : Gain  Gain=12.5  OutDataTypeStr=double
  Mutual Inductor3 : ee_lib/Passive/Transformers/Mutual Inductor  L1=Lm1 H  L2=Lm1/(n^2) H  k=0.99999  L_tol=20  enable_L1_tol=0  L1_tol_distribution=1  L1_nSigma=4  enable_L2_tol=0  L2_tol_distribution=1  L2_nSigma=4  r=[.001, .001] Ohm  g=[1e-09, 1e-09] 1/Ohm  enable_operating_limits=0  operating_limit_action=2  max_working_current=1 A  power_rating=1 W  enable_faults=0  fault_action=1  fault_winding=1  lambdaPercent=50  turnsShort=0  openCct=0  groundShort=0  groundShortG=0 1/Ohm  tau_fault=1e-3 s  enable_temporal_fault=0  t_fault=1 s  enable_behavioral_fault=0  max_permissible_voltage=100 V  n_fail_on_voltage=1  max_permissible_current=1 A  t_fail_on_current=1 s  iL1_specify=off  iL1_priority=High  iL1=0 A  iL1_nominal_specify=off  iL1_nominal_unit=A  iL1_nominal_value=1  iL2_specify=off  iL2_priority=High  iL2=0 A  iL2_nominal_specify=off  iL2_nominal_unit=A  iL2_nominal_value=1
      settings: SourceProductBaseCode=PS  InternalSimscapePortConfiguration="{\"Bottom\":[],\"Left\":[{\"id\":\"p1\",\"label\":\"1+\",\"type\":\"foundation.electrical.electrical\"},{\"id\":\"n1\",\"label\":\"1-\",\"type\":\"foundation.electrical.electrical\"}],\"Right\":[{\"id\":\"p2\",\"label\":\"2+\",\"type\":\"foundation.electrical.electrical\"},{\"id\":\"n2\",\"label\":\"2-\",\"type\":\"foundation.electrical.electrical\"}],\"Top\":[]}"
  Mux5 : Mux  Inputs=2
  Mux6 : Mux  Inputs=2
  PS-Simulink Converter : nesl_utility/PS-Simulink Converter  PhysicalDomain=network_engine_domain  SubClassName=ps_output  LeftPortType=input  RightPortType=output  PseudoPeriodic=off  Frequencies=[]  Unit=inherit  AffineConversion=off
  PS-Simulink Converter{1..2,5..6,20,25,42} (7 alike) : nesl_utility/PS-Simulink Converter  PhysicalDomain=network_engine_domain  SubClassName=ps_output  LeftPortType=input  RightPortType=output  PseudoPeriodic=off  Frequencies=[]  Unit=1  AffineConversion=off
  PS-Simulink Converter3 : nesl_utility/PS-Simulink Converter  Commented=on  PhysicalDomain=network_engine_domain  SubClassName=ps_output  LeftPortType=input  RightPortType=output  PseudoPeriodic=off  Frequencies=[]  Unit=1  AffineConversion=off
  PS-Simulink Converter33 : nesl_utility/PS-Simulink Converter  Commented=on  PhysicalDomain=network_engine_domain  SubClassName=ps_output  LeftPortType=input  RightPortType=output  PseudoPeriodic=off  Frequencies=[]  Unit=1  AffineConversion=off
  PS-Simulink Converter34 : nesl_utility/PS-Simulink Converter  Commented=on  PhysicalDomain=network_engine_domain  SubClassName=ps_output  LeftPortType=input  RightPortType=output  PseudoPeriodic=off  Frequencies=[]  Unit=1  AffineConversion=off
  PS-Simulink Converter4 : nesl_utility/PS-Simulink Converter  PhysicalDomain=network_engine_domain  SubClassName=ps_output  LeftPortType=input  RightPortType=output  PseudoPeriodic=off  Frequencies=[]  Unit=inherit  AffineConversion=off
  Power Sensor : ee_lib/Sensors & Transducers/Power Sensor  measurement_type=2  averaging_period=1e-4 s
      settings: SourceProductBaseCode=PS
  Power Sensor1 : ee_lib/Sensors & Transducers/Power Sensor  measurement_type=2  averaging_period=1e-4 s
      settings: SourceProductBaseCode=PS
  Product{1..7,9} (8 alike) : Product  Commented=on
  Q1P loss : Scope  Commented=on  NumInputPorts=3
  Q1S loss : Scope  Commented=on  NumInputPorts=3
  Q2P loss : Scope  Commented=on  NumInputPorts=3
  Q2S loss : Scope  Commented=on  NumInputPorts=3
  Q3P loss : Scope  Commented=on  NumInputPorts=3
  Q3S loss : Scope  Commented=on  NumInputPorts=3
  Q3S loss1 : Scope
  Q4P loss : Scope  Commented=on  NumInputPorts=3
  Q4S loss : Scope  Commented=on  NumInputPorts=3
  QApri : Subsystem
  QAsec : Subsystem
  QBpri : Subsystem
  QBsec : Subsystem
  QCpri : Subsystem
  QCsec : Subsystem
  QDpri : Subsystem
  QDsec : Subsystem
  Resistor1 : ee_lib/Passive/Resistor  R=0.001 Ohm  R_tol=5  enable_R_tol=0  tol_distribution=1  nSigma=4  enable_operating_limits=0  operating_limit_action=2  max_working_voltage=100 V  power_rating=1 W  enable_faults=0  fault_action=1  R_faulted=inf Ohm  enable_temporal_fault=0  t_fault=1 s  enable_behavioral_fault=0  max_permissible_current=1 A  t_fail_on_current=1 s  noise_mode=0  sample_time=1e-3 s  repeatability=1  auto_seed=1877641321  user_seed=0  Tdevice=25 degC  alpha=3.93e-3 1/K  Tmeas=25 degC  thermal_mass=100 J/K  power_derating_T1=70 degC  power_derating_T2=155 degC  operating_temperature_range_vec=[-50, 150] degC  temperature_specify=off  temperature_priority=High  temperature=298.15 K  temperature_nominal_specify=off  temperature_nominal_unit=K  temperature_nominal_value=1
  Resistor2 : fl_lib/Electrical/Electrical Elements/Resistor  Commented=on  R=1e-3 Ohm  i_specify=off  i_priority=None  i=0 A  i_nominal_specify=off  i_nominal_unit=A  i_nominal_value=1  v_specify=off  v_priority=None  v=0 V  v_nominal_specify=off  v_nominal_unit=V  v_nominal_value=1
  Scope : Scope
  Scope1 : Scope  NumInputPorts=8
  Scope2 : Scope  Commented=on  NumInputPorts=3
  Scope3 : Scope  Commented=on  NumInputPorts=3
  Voltage Sensor{1,3,15,17..18} (5 alike) : fl_lib/Electrical/Electrical Sensors/Voltage Sensor
  Voltage Sensor2 : fl_lib/Electrical/Electrical Sensors/Voltage Sensor  Commented=on
  Voltage Sensor24 : fl_lib/Electrical/Electrical Sensors/Voltage Sensor  Commented=on
  Voltage Sensor25 : fl_lib/Electrical/Electrical Sensors/Voltage Sensor  Commented=on
  iout_total_sense and ocp : Scope  Commented=on  NumInputPorts=2
  llcx_pri_idc : Subsystem  Commented=on
  mult2 : Gain  Gain=0.083
  mult3 : Gain  Gain=0.083
  tank_current_pri : Subsystem  Variant=on
  tank_current_sec : Subsystem  Variant=on
  pri+ : PMIOPort  Side=Left
  sec+ : PMIOPort  Port=2  Side=Right
  sec- : PMIOPort  Port=3  Side=Right
  pri- : PMIOPort  Port=4  Side=Left
  sec_idc : Outport
  pri_idc : Outport  Port=2
  is : Outport  Port=3
  ip : Outport  Port=4
  efficiency : Outport  Port=5
  wires:
  Mux5/1 -> CLLC1: Tank current vs Vsource-source/2  "SEC"
  Product9/1 -> Q1P loss/3
  [Vss_sec] -> mult2/1
  [Itank_pri] -> Mux6/2
  QBpri/1(VDS) -> [QBpri_vds]
  [Vss_pri] -> mult3/1
  Mux6/1 -> CLLC1: Tank current vs Vsource-source/1  "PRI"
  [Itank_sec] -> Mux5/2
  [QBpri_vgs] -> QBpri/1(VGS)
  [QApri_vgs] -> QApri/1(VGS)
  Demux1/1 -> Scope1/1, [QApri_vgs]
  Demux1/2 -> Scope1/2, [QBpri_vgs]
  Demux1/3 -> Scope1/3, [QCpri_vgs]
  Demux1/4 -> Scope1/4, [QDpri_vgs]
  Demux1/8 -> Scope1/8, [QDsec_vgs]
  Demux1/5 -> Scope1/5, [QAsec_vgs]
  Demux1/6 -> Scope1/6, [QBsec_vgs]
  Demux1/7 -> Scope1/7, [QCsec_vgs]
  QApri/2(IDS) -> [QApri_ids]
  QApri/1(VDS) -> [QApri_vds]
  QBpri/2(IDS) -> [QBpri_ids]
  From/1 -> Q1P loss/2, Product9/2
  From1/1 -> Product9/1, Q1P loss/1
  From3/1 -> Q2P loss/1, Product1/1
  From2/1 -> Product1/2, Q2P loss/2
  Product1/1 -> Q2P loss/3
  QCpri/1(VDS) -> [QCpri_vds]
  QCpri/2(IDS) -> [QCpri_ids]
  [QCpri_vgs] -> QCpri/1(VGS)
  [QDpri_vgs] -> QDpri/1(VGS)
  QDpri/2(IDS) -> [QDpri_ids]
  QDpri/1(VDS) -> [QDpri_vds]
  Product2/1 -> Q4P loss/3
  From8/1 -> Q4P loss/2, Product2/2
  From9/1 -> Product2/1, Q4P loss/1
  From7/1 -> Q3P loss/1, Product3/1
  From6/1 -> Product3/2, Q3P loss/2
  Product3/1 -> Q3P loss/3
  PS-Simulink Converter34/1 -> iout_total_sense and ocp/2
  PS-Simulink Converter33/1 -> iout_total_sense and ocp/1
  [QCsec_vgs] -> QCsec/1(VGS)
  QCsec/2(IDS) -> [QCsec_ids]
  QCsec/1(VDS) -> [QCsec_vds]
  QDsec/1(VDS) -> [QDsec_vds]
  QDsec/2(IDS) -> [QDsec_ids]
  [QDsec_vgs] -> QDsec/1(VGS)
  [QBsec_vgs] -> QBsec/1(VGS)
  QBsec/2(IDS) -> [QBsec_ids]
  QBsec/1(VDS) -> [QBsec_vds]
  QAsec/1(VDS) -> [QAsec_vds]
  QAsec/2(IDS) -> [QAsec_ids]
  [QAsec_vgs] -> QAsec/1(VGS)
  Product6/1 -> Q3S loss/3
  From19/1 -> Q3S loss/2, Product6/2
  From20/1 -> Product6/1, Q3S loss/1
  From22/1 -> Q4S loss/1, Product5/1
  From21/1 -> Product5/2, Q4S loss/2
  Product5/1 -> Q4S loss/3
  Product4/1 -> Q2S loss/3
  From16/1 -> Q2S loss/2, Product4/2
  From18/1 -> Product4/1, Q2S loss/1
  From15/1 -> Q1S loss/1, Product7/1
  From14/1 -> Product7/2, Q1S loss/2
  Product7/1 -> Q1S loss/3
  PS-Simulink Converter20/1 -> [CR1_V]
  tank_current_pri/1(to_scope) -> [Itank_pri], ip/1
  tank_current_sec/1(to_scope) -> [Itank_sec], is/1
  mult3/1 -> Mux6/1
  mult2/1 -> Mux5/1
  PS-Simulink Converter2/1 -> Scope/1
  pwm/1 -> Multiply2/1
  Multiply2/1 -> Demux1/1
  PS-Simulink Converter/1 -> [llc1_pri_pave]
  PS-Simulink Converter4/1 -> [llc1_sec_pave]
  [llc1_sec_pave] -> Display/1, Divide/1
  [llc1_pri_pave] -> Display1/1, Divide/2
  Divide/1 -> efficiency/1
  From28/1 -> Scope2/3
  From27/1 -> Scope2/2
  From24/1 -> Scope2/1
  From29/1 -> Scope3/1
  From30/1 -> Scope3/2
  From31/1 -> Scope3/3
  PS-Simulink Converter3/1 -> ?
  PS-Simulink Converter5/1 -> First-Order Filter/1
  First-Order Filter/1 -> pri_idc/1
  PS-Simulink Converter25/1 -> [Vss_pri]
  PS-Simulink Converter1/1 -> [CR2_V]
  PS-Simulink Converter6/1 -> [Vss_sec]
  PS-Simulink Converter42/1 -> sec_idc/1, Q3S loss1/1
  connections:
  pri-/RConn1 -- Power Sensor/LConn3 -- QBpri/LConn2 -- QDpri/LConn2 -- Capacitor3/RConn1
  PS-Simulink Converter20/LConn1 -- Voltage Sensor15/RConn1
  Mutual Inductor3/RConn2 -- tank_current_sec/LConn1
  Voltage Sensor15/LConn1 -- CrP1/LConn1 -- Voltage Sensor17/LConn1 -- QCpri/LConn2 -- QDpri/LConn1
  Power Sensor1/LConn3 -- sec-/RConn1 -- Capacitor2/RConn1 -- QBsec/LConn2 -- QDsec/LConn2
  Mutual Inductor3/LConn2 -- tank_current_pri/LConn2
  Current Sensor8/LConn1 -- Resistor1/RConn1
  PS-Simulink Converter42/LConn1 -- Current Sensor8/RConn1
  Current Sensor8/RConn2 -- Power Sensor1/LConn2
  QApri/LConn2 -- tank_current_pri/LConn1 -- Voltage Sensor17/RConn2 -- QBpri/LConn1
  Current+OCP sense/RConn2 -- Voltage Sensor24/RConn2
  PS-Simulink Converter34/LConn1 -- Voltage Sensor25/RConn1
  PS-Simulink Converter33/LConn1 -- Voltage Sensor24/RConn1
  Current+OCP sense/RConn1 -- Voltage Sensor24/LConn1
  Current+OCP sense/RConn4 -- Voltage Sensor25/RConn2
  Current+OCP sense/RConn3 -- Voltage Sensor25/LConn1
  Voltage Sensor18/RConn1 -- PS-Simulink Converter1/LConn1
  Voltage Sensor1/RConn1 -- PS-Simulink Converter2/LConn1
  Power Sensor/LConn2 -- pri+/RConn1
  QCpri/LConn1 -- Capacitor3/LConn1 -- Current Sensor/LConn1 -- QApri/LConn1
  PS-Simulink Converter/LConn1 -- Power Sensor/RConn1
  PS-Simulink Converter4/LConn1 -- Power Sensor1/RConn1
  Voltage Sensor1/RConn2 -- LrP1/LConn1 -- CrP1/RConn1 -- Voltage Sensor15/RConn2 -- Voltage Sensor1/LConn1
  LrP1/RConn1 -- Mutual Inductor3/LConn1
  Resistor1/LConn1 -- QCsec/LConn1 -- QAsec/LConn1 -- Capacitor2/LConn1
  Resistor2/RConn1 -- llcx_pri_idc/LConn2
  Voltage Sensor2/RConn2 -- llcx_pri_idc/RConn2
  Voltage Sensor2/LConn1 -- llcx_pri_idc/RConn1
  PS-Simulink Converter3/LConn1 -- Voltage Sensor2/RConn1
  Resistor2/LConn1 -- llcx_pri_idc/LConn1
  Current Sensor/RConn2 -- Power Sensor/LConn1
  PS-Simulink Converter5/LConn1 -- Current Sensor/RConn1
  sec+/RConn1 -- Power Sensor1/LConn1
  Voltage Sensor17/RConn1 -- PS-Simulink Converter25/LConn1
  LrS1/LConn1 -- Mutual Inductor3/RConn1
  Voltage Sensor3/RConn1 -- PS-Simulink Converter6/LConn1
  Voltage Sensor18/RConn2 -- CrS1/RConn1 -- QDsec/LConn1 -- QCsec/LConn2 -- Voltage Sensor3/LConn1
  Voltage Sensor3/RConn2 -- tank_current_sec/LConn2 -- QBsec/LConn1 -- QAsec/LConn2
  Voltage Sensor18/LConn1 -- CrS1/LConn1 -- LrS1/RConn1
